simulink model "controller13_AIS"  (R2020b)
settings: Solver=FixedStepDiscrete  StartTime=0.0  StopTime=inf  RelTol=1e-3
values from neighbouring files (symbols this model uses):
  ctr = make_controller()    [setup_controller_with_functions.m]
  mdl = make_model(flight_time)    [setup_controller_with_functions.m]
  ukf_P0_flat = UKF.flatten_matrix(ukf_sys.P0)    [controller_setup_ukf.m]
  ukf_prediction_time = 0.015    [controller_setup_ukf.m]
  ukf_s0 = ukf_sys.s0    [controller_setup_ukf.m]
  ukf_sys = UKF.initialize_ukf_sys(rbt, mdl, ukf_params)    [controller_setup_ukf.m]
  ukf_use_prediction = 1    [controller_setup_ukf.m]
undefined symbols (not defined in the file or in its folder): ctr1, ctr2, DiscIntNeverNeededParam, flt, IO397, rbt1, rbt2, rsim1, rsim2, som, traj2
libraries: simulink x63, slrealtimeloglib x21, slrealtimetgmanagement x8, slrealtimeseriallib x5, speedgoatlib_fpga_analog_io x4, slrealtimeutilitieslib x3, dspfdesign x2, speedgoatlib_fpga x2, slrealtimeiplib x2, speedgoatlib_fpga_dio x1
(part 5 of 5)

== matlab function controller13_AIS/Adaptive Controller 1/somersault_phase ==
  data: som_phase output; time input; mdl parameter; som parameter
function som_phase  = fcn(time, mdl, som)
%#codegen

som_phase = 0;  % during a normal flight
if som.en
    if time > som.t_start + som.t_rise + som.t_acc + som.t_dcc + som.t_rec
        som_phase = 0;  % afterwards
    elseif time > som.t_start + som.t_rise + som.t_acc + som.t_dcc
        som_phase = 4;  % recovery
    elseif time > som.t_start + som.t_rise + som.t_acc
        som_phase = 3;  % rolling, second half.
    elseif time > som.t_start + som.t_rise
        som_phase = 2;  % rolling, first half.
    elseif time > som.t_start
        som_phase = 1;  % gaining altitude
    end
end

== matlab function controller13_AIS/Force//Torque to Trajectory Specs 1/nominal desired voltage/force to voltage flipping/MATLAB Function ==
  data: Vi input; Vo output; ctr1 parameter
function Vo = fcn(Vi,ctr1)
%old script
% if max(Vi)>mdl.max_v
%     Vo = Vi * mdl.max_v/max(Vi);
%     % scale down all votages if one exceeds the max limit.
% else
%     Vo = Vi;
% end

%new change (modify max_v to a vector so each DEA has its own max)
scale_down_ratio_vec = Vi ./ ctr1.safety.volt;
scale_down_ratio = max(scale_down_ratio_vec);
bool_scale_down = scale_down_ratio>1;

if bool_scale_down
   Vo = Vi/scale_down_ratio;
else
   Vo = Vi; 
end

== matlab function controller13_AIS/smothing 1/smoothing ==
  data: time input; out_amp output; amp input; amp2 input; som parameter
function out_amp  = fcn(time,amp,amp2,som)
%#codegen

alp = 1;
if time > som.t_start + som.t_rise + som.t_acc + som.t_dcc + som.t_rec
    alp = 1;  % afterwards
elseif time > som.t_start
    alp = som.filter.alp;
end
% set en = 0 if the robot goes out of the safe envelope.
out_amp = som.filter.alp*amp + (1-som.filter.alp)*amp2;

== matlab function controller13_AIS/Adaptive Controller 1/saturation ==
  data: x_roll input; X_roll output size=1; y_pitch input; z_yaw input; Y_pitch output size=1; Z_yaw output size=1; Th input; Force output size=1; rbt1 parameter; ctr1 parameter; som_phase input; som parameter
function [X_roll, Y_pitch, Z_yaw, Force] = fcn(x_roll, y_pitch, z_yaw, Th, rbt1, ctr1, som_phase, som)
%#codegen

X_roll = max(min(x_roll, ctr1.lim.taux), -ctr1.lim.taux);
%X_roll = x_roll;
Y_pitch = max(min(y_pitch, ctr1.lim.tauy), -ctr1.lim.tauy);
%Y_pitch = y_pitch;
Z_yaw = max(min(z_yaw, ctr1.lim.tauz), -ctr1.lim.tauz);

Force = Th*rbt1.m;

% F is already checked for saturation, but still needs to be converted into
% Newton

%% Roll torque management (somersault)
if som_phase == 2
    X_roll = som.roll_mag; % torque in SI
    Y_pitch = 0;  % to turn of the pitch control
elseif som_phase == 3
    X_roll = -som.roll_mag; % torque in SI
    Y_pitch = 0;  % to turn of the pitch control
end
    
%% Thrust management
% thrust is not controlled during the flipping maneuver (the output here will be overridden in the mapping).

== matlab function controller13_AIS/Force//Torque to Trajectory Specs 1/force//torque to module thrust/mapping scheme (flipping compataible) ==
  data: time input; module_f output; inputs input; rbt1 parameter; som parameter; mdl parameter
function module_f  = fcn(time, inputs, rbt1, som, mdl)

% somersault
if som.en
    if time > som.t_start + som.t_rise + som.t_acc + som.t_dcc+som.t_rec % after recovery
        %
    elseif time > som.t_start + som.t_rise + som.t_acc + som.t_dcc % recovery
        %inputs(1) = rbt.m*(mdl.g*(som.thrust_f+0.2));
    elseif time > som.t_start + som.t_rise % rolling, first half+second half.
        % priortize the roll torque and ensure non-negative forces.
        inputs(1) = 0;
    elseif time > som.t_start
        inputs(1) = rbt1.m*(mdl.g*som.thrust_f); % during the t rise.                
    end
end

% torque/thrust to unit force mapping
if rbt1.til == 0
    module_f = rbt1.Apinv * inputs(1:3); % original mapping
elseif rbt1.til > 0
    module_f = rbt1.A2inv * inputs;
else
    module_f = [0 0 0 0]';
end

% safety
if min(module_f) < 0
    module_f = module_f - min(module_f); % this ensure positive module forces
end

end

== matlab function controller13_AIS/Adaptive Controller 1/adaptive system/integrator/initial guess ==
  data: i_e input; int_e output; tor_off input; th_off input; tor_inte output; th_inte output; ctr1 parameter; rbt1 parameter; mdl parameter
function [int_e, tor_inte, th_inte] = fcn(i_e, tor_off, th_off, ctr1, rbt1, mdl)
%#codegen

tor_inte = zeros(3,1);
int_e    = zeros(4,1);

int_e(1) = i_e(1)+tor_off(1);
int_e(2) = i_e(2)+tor_off(2);
int_e(3) = i_e(3)+tor_off(3);
int_e(4) = i_e(4)+th_off;

tor_inte(1) = int_e(1)*ctr1.gain.ati*rbt1.ixx/mdl.g;
tor_inte(2) = int_e(2)*ctr1.gain.ati*rbt1.iyy/mdl.g;
tor_inte(3) = 0;

th_inte     = int_e(4)*ctr1.gain.ali;

== matlab function controller13_AIS/Phantom trigger/start at one ==
  data: time input; trigger output
function trigger = fcn(time)
%#codegen
trigger = 0;
if time > 1
   trigger = 1; 
end
if time > 2
   trigger = 0; 
end

== matlab function controller13_AIS/Measurement manager 1/safety check system/envelope check ==
  data: x input; en output; y input; z input; ctr1 parameter
function en  = fcn(x,y,z, ctr1)

if abs(x)>ctr1.safety.enableZone.xmax || abs(y)>ctr1.safety.enableZone.ymax || abs(z)>ctr1.safety.enableZone.zmax
    en = 0;
else
    en = 1;
end

end

== matlab function controller13_AIS/Dynamic Sim 1/conditioning ==
  data: Rout output; Rin input; eu output
function [Rout, eu]  = fcn(Rin)
%#codegen
Rm = [Rin(1:3)./norm(Rin(1:3)),Rin(4:6)./norm(Rin(4:6)),Rin(7:9)./norm(Rin(7:9))];
% conditioning on orthogonality.
Rout = [Rm(:,1);Rm(:,2);Rm(:,3)];

% euler angles
euy = asin(min(max(Rm(1,3),-1),1));
eux = atan2(-Rm(2,3),Rm(3,3));
euz = atan2(-Rm(1,2),Rm(1,1));
%euz=acos(min(max(Rm(1,1)/cos(euy),-1),1));
%eux=acos(min(max(Rm(3,3)/cos(euy),-1),1));
eu = [eux;euy;euz];
% not being very careful with singularities.

== matlab function controller13_AIS/Force//Torque to Trajectory Specs 1/nominal desired voltage/map_selection ==
  data: hover_map output; time input; mdl parameter; som parameter
function hover_map  = fcn(time, mdl, som)
%#codegen

hover_map = 1;  % during a normal flight
if som.en
    if time > som.t_start + som.t_rise + som.t_acc + som.t_dcc
        hover_map = 1;  % afterwards
    elseif time > som.t_start + som.t_rise
    %elseif time > som.t_start + som.t_rise 
        hover_map = 0;  % 
    end
end

== matlab function controller13_AIS/Dynamic Sim 1/rigid body dynamics sim ==
  data: dv output double size=3; mforces input double; dR output double size=9; dw output double size=3; v input; R input; w input; rbt1 parameter; mdl parameter; disturbance input; rsim1 parameter
function [dv, dR, dw]  = fcn(mforces,v,R,w,rbt1,mdl,disturbance, rsim1)
%#codegen

% noiseless
% no damping
% rbt_A_temp = [rbt.A; 0.015 -0.015 0.015 -0.015];
rbt_A_temp = rbt1.A2;
% inputs = rbt.A * mforces(:);
inputs = rbt_A_temp * mforces(:);
thrust = inputs(1);
% torque = [inputs(2);inputs(3);0];
torque = [inputs(2);inputs(3);inputs(4)];
%R = R(:);
%w = w(:);
dv = R(7:9)*thrust/rbt1.m - [0;0;mdl.g] + disturbance(1:3);

dw = diag([rsim1.rbt.ixx, rsim1.rbt.iyy, rsim1.rbt.izz]) \ ( (torque) - cross(w,diag([rsim1.rbt.ixx, rsim1.rbt.iyy, rsim1.rbt.izz])*w)+ disturbance(4:6) ) ;
dR1 = R(4:6)*w(3)-R(7:9)*w(2);
dR2 = R(7:9)*w(1)-R(1:3)*w(3);
dR3 = R(1:3)*w(2)-R(4:6)*w(1);
dR = [dR1;dR2;dR3];
%dv = zeros(3,1);
%dw = zeros(3,1);
%dR = zeros(9,1);

== matlab function controller13_AIS/Adaptive Controller 1/attitude and thrust controller/Yaw Controller/desired yaw ==
  data: t input; id input; rd_yaw output; ctr1 parameter; index output; mdl parameter
function [rd_yaw, index] = fcn(t,id,ctr1,mdl)

if ctr1.yaw.dy.en
    
    if id > 1
        t_cum = sum(ctr1.yaw.dy.duration(1:id-1))+sum(ctr1.yaw.dy.trans(1:id-1));
    else
        t_cum = 0;
    end

    if t > mdl.i_delay + t_cum && t <= mdl.i_delay + t_cum + ctr1.yaw.dy.duration(id)
        rd_yaw = ctr1.yaw.dy.angle(id);
    elseif t > mdl.i_delay + t_cum + ctr1.yaw.dy.duration(id) && t < mdl.i_delay + t_cum + ctr1.yaw.dy.duration(id) + ctr1.yaw.dy.trans(id)
        rd_yaw = ctr1.yaw.dy.angle(id) + (ctr1.yaw.dy.angle(id+1)-ctr1.yaw.dy.angle(id))/ctr1.yaw.dy.trans(id)*(t-mdl.i_delay-t_cum-ctr1.yaw.dy.duration(id));
    elseif t >= mdl.i_delay + t_cum + ctr1.yaw.dy.duration(id) + ctr1.yaw.dy.trans(id)
        rd_yaw = ctr1.yaw.dy.angle(id+1);
        id = id + 1;
    else
        rd_yaw = 0;
    end

else
    
    rd_yaw = ctr1.setpoint.yaw;
    
end

index = id;
    
end

== matlab function controller13_AIS/Measurement manager 1/safety check system/voltage check ==
  data: voltage input; en output; ctr1 parameter
function en  = fcn(voltage, ctr1)

if sum(voltage>ctr1.safety.volt) > 0
    en = 0;
else
    en = 1;
end

end

== matlab function controller13_AIS/Measurement manager 1/envelope//voltage check ==
  data: x input; keep_flying output size=1; y input; z input; ctr1 parameter
function keep_flying  = fcn(x,y,z,ctr1)

if abs(x)>ctr1.safety.land.xmax || abs(y)>ctr1.safety.land.ymax || abs(z)>ctr1.safety.land.zmax
    keep_flying = 0;
% elseif voltage(1) > ctr.safety.land.volt
%     keep_flying = 0;    
else
    keep_flying = 1;
end

end

== matlab function controller13_AIS/Measurement manager 1/MATLAB Function ==
  data: keep_flying input; landing_in input; landing_out output size=1; cum_in input; cum_out output size=1; ctr1 parameter; mdl parameter
function [landing_out, cum_out] = fcn(keep_flying, landing_in, cum_in, ctr1, mdl)

if keep_flying == 0
    cum_out = cum_in + mdl.T;
else
    cum_out = 0;
end

if cum_out > ctr1.safety.land.T || landing_in == 1
    landing_out = 1;
else 
    landing_out = 0;
end

end

== matlab function controller13_AIS/Measurement manager 1/voltage check ==
  data: voltage input; keep_flying output size=1; ctr1 parameter
function keep_flying  = fcn(voltage, ctr1)

% if voltage(1)>ctr.safety.land.volt || voltage(2)>ctr.safety.land.volt || voltage(3)>ctr.safety.land.volt || voltage(4)>ctr.safety.land.volt

if sum(voltage>ctr1.safety.land.volt)>0
    keep_flying = 0;
else
    keep_flying = 1;
end

end

== matlab function controller13_AIS/Measurement manager 1/safety check system/MATLAB Function ==
  data: keep_flying input; en_in input; en_out output size=1; cum_in input; cum_out output size=1; ctr1 parameter; mdl parameter
function [en_out, cum_out] = fcn(keep_flying, en_in, cum_in, ctr1, mdl)

if keep_flying == 0
    cum_out = cum_in + mdl.T;
else
    cum_out = 0;
end

if cum_out > ctr1.safety.T || en_in == 0
    en_out = 0;
else 
    en_out = 1;
end

end

== matlab function controller13_AIS/MATLAB Function ==
  data: u input; y output
function y = fcn(u)

y = u;

== matlab function controller13_AIS/Adaptive Controller 1/attitude and thrust controller/External Torque Observer ==
  data: omega input; omega_hat output; torque_x input; torque_y input; torque_z input; ext_torque_hat input; omega_hat input; time input; ext_torque_hat output; ctr1 parameter; rbt1 parameter; mdl parameter
function [omega_hat, ext_torque_hat] = fcn(omega, torque_x, torque_y, torque_z, ext_torque_hat, omega_hat, time, ctr1, rbt1, mdl)
    
omega_hat           = omega_hat(:);
ext_torque_hat      = ext_torque_hat(:);
J                   = diag([rbt1.ixx, rbt1.iyy, rbt1.izz]);
omega_cross_J_omega = cross(omega, J*omega);
x_hat_curr          = diag(ctr1.torque_obs.state_scaling)*[omega_hat(:); ext_torque_hat(:)];

% til = 20;

if rbt1.til == 0
    u              = diag(ctr1.torque_obs.input_scaling)*[torque_x - omega_cross_J_omega(1); torque_y - omega_cross_J_omega(2)];
    y              = diag(ctr1.torque_obs.meas_scaling)*omega(1:2); 
    x_hat_pred     = ctr1.torque_obs.A*x_hat_curr + ctr1.torque_obs.B(:, 1:2)*u; 
    x_hat_next     = diag(ctr1.torque_obs.out_scaling)*(x_hat_pred + ctr1.torque_obs.L*(y - ctr1.torque_obs.C*x_hat_pred));
    omega_hat      = x_hat_next(1:2,1);
    ext_torque_hat = x_hat_next(3:4,1);
    if time < mdl.i_delay
        omega_hat      = zeros(2,1);
        ext_torque_hat = zeros(2,1);
    end
else
    u              = diag(ctr1.torque_obs.input_scaling)*[torque_x - omega_cross_J_omega(1); torque_y - omega_cross_J_omega(2); torque_z - omega_cross_J_omega(3)];
    y              = diag(ctr1.torque_obs.meas_scaling)*omega(1:3); 
    x_hat_pred     = ctr1.torque_obs.A*x_hat_curr + ctr1.torque_obs.B(:, 1:3)*u; 
    x_hat_next     = diag(ctr1.torque_obs.out_scaling)*(x_hat_pred + ctr1.torque_obs.L*(y - ctr1.torque_obs.C*x_hat_pred));
    omega_hat      = x_hat_next(1:3,1);
    ext_torque_hat = x_hat_next(4:6,1);
    if time < mdl.i_delay
        omega_hat      = zeros(3,1);
        ext_torque_hat = zeros(3,1);
    end
end



end

== matlab function controller13_AIS/Adaptive Controller 2/adaptive setpoint rd ==
  data: rd output; rd_d output; rd_dd output; rd_ddd output; rd_dddd output; time input; r input; r_d input; landing input; som_ph input; id_in input; ctr2 parameter; som parameter; mdl parameter; traj2 parameter; id_out output
function [rd,rd_d,rd_dd,rd_ddd,rd_dddd,id_out] = fcn(time, r, r_d, landing, som_ph, id_in, ctr2, som, mdl, traj2)
%#codegen

rd = [ctr2.setpoint.x; ctr2.setpoint.y; ctr2.setpoint.z];
rd_d = zeros(3,1);
rd_dd = zeros(3,1);
rd_ddd = zeros(3,1);
rd_dddd = zeros(3,1);

if time <= mdl.i_delay+0.1
    rd_z = ctr2.takeoff.height;
    rd   = [ctr2.setpoint.x; ctr2.setpoint.y; rd_z];
end

% takeoff
if ctr2.takeoff.en
    if time > mdl.i_delay+0.1 && time < (mdl.i_delay+0.1+ctr2.takeoff.time)
        
        % rd_z (desired position)
        rd_z = ctr2.takeoff.height + (((ctr2.setpoint.z-ctr2.takeoff.height)/ctr2.takeoff.time)*(time-mdl.i_delay-0.1));
        if rd_z > ctr2.setpoint.z
            rd_z = ctr2.setpoint.z;
        end
        rd   = [ctr2.setpoint.x; ctr2.setpoint.y; rd_z];
        
        % rd_d_z (desired velocity)
        rd_d_z = ((ctr2.setpoint.z-ctr2.takeoff.height)/ctr2.takeoff.time);
        rd_d   = [rd_d(1); rd_d(2); rd_d_z];
        
    end
end

% planned landing 
if ctr2.landing.en
    if time > (mdl.rt-ctr2.landing.time)
        
        % rd_z (desired position)
        rd_z = ctr2.setpoint.z-(((ctr2.setpoint.z-ctr2.landing.height)/ctr2.landing.time)*(time-mdl.rt+ctr2.landing.time));
        if rd_z < ctr2.landing.height
            rd_z = ctr2.landing.height;
        end
        rd   = [ctr2.setpoint.x; ctr2.setpoint.y; rd_z];
        
        % rd_d_z (desired velocity)
        rd_d_z = (ctr2.landing.height-ctr2.setpoint.z)/ctr2.landing.time;
        rd_d   = [rd_d(1); rd_d(2); rd_d_z];
        
    end
end

% forced landing
if landing
    rd_z = 0.02;
    rd   = [ctr2.setpoint.x; ctr2.setpoint.y; rd_z];
end


% somersault
if som.en
    if time > som.t_start + som.t_rise + som.t_acc + som.t_dcc + som.t_rec
        % % afterwards 
        %dt = som.t_start + som.t_rise + som.t_acc + som.t_dcc + som.t_rec - time;
        %rd = rd + dt*(r-rd);
    elseif time > som.t_start + som.t_rise + som.t_acc + som.t_dcc
        % recovery
        dt = som.t_start + som.t_rise + som.t_acc + som.t_dcc + som.t_rec - time;
        rd = rd + (dt/som.t_rec)*(r-rd);
        rd_d = rd_d + 0.5*(dt/som.t_rec)*(r_d-rd_d);
        rd(1) = min(max(rd(1),-0.25),0.25); % 25 cm envelope
        rd(2) = min(max(rd(2),-0.25),0.25); % 25 cm envelope
        rd(3) = max(rd(3),0.02); % min altitude setpoint.
    end
end

% update id for predefined trajectory
id      = floor(id_in);
id_out  = id_in + 1;

% use predefined trajectory
if traj2.en
    rd      = traj2.origin + traj2.rd(1:3,id);
    rd_d    = traj2.rd_d(1:3,id);
    rd_dd   = traj2.rd_dd(1:3,id);
    rd_ddd  = traj2.rd_ddd(1:3,id);
    rd_dddd = traj2.rd_dddd(1:3,id);
end



end

== matlab function controller13_AIS/Adaptive Controller 1/attitude and thrust controller/Yaw Controller/MATLAB Function ==
  data: torq_ext input; torq_z input; torq_z output; ctr1 parameter; rbt1 parameter
function torq_z = fcn(torq_ext,torq_z,ctr1, rbt1)

% if rbt1.til > 0
%     if ctr1.yaw.dy.en == 0
%         torq_z = torq_z - torq_ext(3) * ctr1.torque_obs.factor.z;
%     end
% end

end

== matlab function controller13_AIS/Adaptive Controller 2/adaptive system/integrator/initial guess ==
  data: i_e input; int_e output; tor_off input; th_off input; tor_inte output; th_inte output; ctr2 parameter; rbt2 parameter; mdl parameter
function [int_e, tor_inte, th_inte] = fcn(i_e, tor_off, th_off, ctr2, rbt2, mdl)
%#codegen

tor_inte = zeros(3,1);
int_e    = zeros(4,1);

int_e(1) = i_e(1)+tor_off(1);
int_e(2) = i_e(2)+tor_off(2);
int_e(3) = i_e(3)+tor_off(3);
int_e(4) = i_e(4)+th_off;

tor_inte(1) = int_e(1)*ctr2.gain.ati*rbt2.ixx/mdl.g;
tor_inte(2) = int_e(2)*ctr2.gain.ati*rbt2.iyy/mdl.g;
tor_inte(3) = 0;

th_inte     = int_e(4)*ctr2.gain.ali;

== matlab function controller13_AIS/Adaptive Controller 2/attitude and thrust controller/Attitude Controleller ==
  data: r input; torque_x output size=1; r_dot input; r_dotdot input; R input; Omega input; rd input; rd_d input; rd_dd input; rd_ddd input; rd_dddd input; int_e input; ext_torq input; ctr2 parameter; rbt2 parameter; torque_y output size=1; torque_z output size=1; att_e output size=3; mdl parameter
 function [torque_x, torque_y, torque_z, att_e] = fcn(r, r_dot, r_dotdot, R, Omega, rd,rd_d,rd_dd,rd_ddd,rd_dddd, int_e, ext_torq, ctr2, rbt2, mdl)
%#codegen

%% init
R11 = R(1);
R12 = R(2);
R13 = R(3);
R21 = R(4);
R22 = R(5);
R23 = R(6);
R31 = R(7);
R32 = R(8);
R33 = R(9);
R1 = [R11; R21; R31];     % unit (column) vector
R2 = [R12; R22; R32];
R3 = [R13; R23; R33];
wx = Omega(1);
wy = Omega(2);
wz = Omega(3);

Dr = r-rd;
Dr_dot = r_dot-rd_d;

torque_x = -dot(R2,rd_dddd) - ...
    ctr2.gain.at3*( mdl.g*wx+dot(R2,rd_ddd) ) - ...
    ctr2.gain.at2*( dot(R2,mdl.g*[0;0;1]+rd_dd) ) + ...
    ctr2.gain.at1*( dot(R2,Dr_dot) ) + ...
    ctr2.gain.at0*( dot(R2,Dr) ) + ...
    ctr2.gain.ati*( int_e(1) );
torque_x = torque_x*rbt2.ixx/mdl.g - ext_torq(1)*ctr2.torque_obs.factor.x;

torque_y = dot(R1,rd_dddd) - ...
    ctr2.gain.at3*( mdl.g*wy-dot(R1,rd_ddd) ) - ...
    ctr2.gain.at2*( dot(R1,-mdl.g*[0;0;1]-rd_dd) ) - ...
    ctr2.gain.at1*( dot(R1,Dr_dot) ) - ...
    ctr2.gain.at0*( dot(R1,Dr) ) + ...
    ctr2.gain.ati*( int_e(2) );

torque_y = torque_y*rbt2.iyy/mdl.g - ext_torq(2)*ctr2.torque_obs.factor.y;

torque_z = 0;           % no yaw control

att_e = -[-dot(R2,Dr);dot(R1,Dr);0];

== matlab function controller13_AIS/Adaptive Controller 1/observer/Rotaion/Rotation Matrix1 ==
  data: R input; Rdot input; w output
function w  = fcn(R,Rdot)
%#codegen
w = zeros(3,1);
w(1) = R(3)*Rdot(2) + R(6)*Rdot(5) + R(9)*Rdot(8);
w(2) = R(1)*Rdot(3) + R(4)*Rdot(6) + R(7)*Rdot(9);
w(3) = R(2)*Rdot(1) + R(5)*Rdot(4) + R(8)*Rdot(7);

% w = R^T * dot(R)

end

== matlab function controller13_AIS/Adaptive Controller 2/attitude and thrust controller/External Torque Observer ==
  data: omega input; omega_hat output; torque_x input; torque_y input; torque_z input; ext_torque_hat input; omega_hat input; time input; ext_torque_hat output; ctr2 parameter; rbt2 parameter; mdl parameter
function [omega_hat, ext_torque_hat] = fcn(omega, torque_x, torque_y, torque_z, ext_torque_hat, omega_hat, time, ctr2, rbt2, mdl)
    
omega_hat           = omega_hat(:);
ext_torque_hat      = ext_torque_hat(:);
J                   = diag([rbt2.ixx, rbt2.iyy, rbt2.izz]);
omega_cross_J_omega = cross(omega, J*omega);
x_hat_curr          = diag(ctr2.torque_obs.state_scaling)*[omega_hat(:); ext_torque_hat(:)];

% til = 20;

if rbt2.til == 0
    u              = diag(ctr2.torque_obs.input_scaling)*[torque_x - omega_cross_J_omega(1); torque_y - omega_cross_J_omega(2)];
    y              = diag(ctr2.torque_obs.meas_scaling)*omega(1:2); 
    x_hat_pred     = ctr2.torque_obs.A*x_hat_curr + ctr2.torque_obs.B(:, 1:2)*u; 
    x_hat_next     = diag(ctr2.torque_obs.out_scaling)*(x_hat_pred + ctr2.torque_obs.L*(y - ctr2.torque_obs.C*x_hat_pred));
    omega_hat      = x_hat_next(1:2,1);
    ext_torque_hat = x_hat_next(3:4,1);
    if time < mdl.i_delay
        omega_hat      = zeros(2,1);
        ext_torque_hat = zeros(2,1);
    end
else
    u              = diag(ctr2.torque_obs.input_scaling)*[torque_x - omega_cross_J_omega(1); torque_y - omega_cross_J_omega(2); torque_z - omega_cross_J_omega(3)];
    y              = diag(ctr2.torque_obs.meas_scaling)*omega(1:3); 
    x_hat_pred     = ctr2.torque_obs.A*x_hat_curr + ctr2.torque_obs.B(:, 1:3)*u; 
    x_hat_next     = diag(ctr2.torque_obs.out_scaling)*(x_hat_pred + ctr2.torque_obs.L*(y - ctr2.torque_obs.C*x_hat_pred));
    omega_hat      = x_hat_next(1:3,1);
    ext_torque_hat = x_hat_next(4:6,1);
    if time < mdl.i_delay
        omega_hat      = zeros(3,1);
        ext_torque_hat = zeros(3,1);
    end
end



end

== matlab function controller13_AIS/Adaptive Controller 2/attitude and thrust controller/Thrust Controller ==
  data: r input; F output size=1; r_dot input; r_dotdot input; R input; Omega input; rd input; rd_d input; rd_dd input; rd_ddd input; rd_dddd input; int_e input; mdl parameter; alt_e output size=1; ctr2 parameter
function [F, alt_e] = fcn(r, r_dot, r_dotdot, R, Omega, rd,rd_d,rd_dd,rd_ddd,rd_dddd, int_e, mdl, ctr2)
%#codegen

%% init
R11 = R(1);
R12 = R(2);
R13 = R(3);
R21 = R(4);
R22 = R(5);
R23 = R(6);
R31 = R(7);
R32 = R(8);
R33 = R(9);

% feedforward
% -> (0m, 0) -> (0.1m, 0.2)
ffwd = mdl.g * max(0,(rd(3)*1.25-ctr2.takeoff.height));

F = rd_dd(3) - ctr2.gain.al1*( r_dot(3)-rd_d(3) ) - ctr2.gain.al0*( r(3)-rd(3) );
% F = 0 - ctr.gain.al1*( r_dot(3)) - ctr.gain.al0*( r(3)-ctr.setpoint.z );
F = mdl.g + F + ctr2.gain.ali*int_e(4) + ffwd; % g + control + integral + feedforward
F = F/R33;
F = max(min(F, mdl.g+4), mdl.g-4.0); % during hovering.

alt_e = -( r(3)-rd(3) )/R33;
% alt_e = -( r(3)- ctr.setpoint.z )/R33;
end

== matlab function controller13_AIS/Adaptive Controller 2/attitude and thrust controller/Yaw Controller/MATLAB Function ==
  data: torq_ext input; torq_z input; torq_z output; ctr2 parameter; rbt2 parameter
function torq_z = fcn(torq_ext,torq_z,ctr2, rbt2)

if rbt2.til > 0
    if ctr2.yaw.dy.en == 0
%         torq_z = torq_z - torq_ext(3) * ctr2.torque_obs.factor.z;
    end
else
    torq_z = torq_z;
end

end

== matlab function controller13_AIS/Adaptive Controller 2/attitude and thrust controller/Yaw Controller/desired yaw ==
  data: t input; id input; rd_yaw output; ctr2 parameter; index output; mdl parameter
function [rd_yaw, index] = fcn(t,id,ctr2,mdl)

if ctr2.yaw.dy.en
    
    if id > 1
        t_cum = sum(ctr2.yaw.dy.duration(1:id-1))+sum(ctr2.yaw.dy.trans(1:id-1));
    else
        t_cum = 0;
    end

    if t > mdl.i_delay + t_cum && t <= mdl.i_delay + t_cum + ctr2.yaw.dy.duration(id)
        rd_yaw = ctr2.yaw.dy.angle(id);
    elseif t > mdl.i_delay + t_cum + ctr2.yaw.dy.duration(id) && t < mdl.i_delay + t_cum + ctr2.yaw.dy.duration(id) + ctr2.yaw.dy.trans(id)
        rd_yaw = ctr2.yaw.dy.angle(id) + (ctr2.yaw.dy.angle(id+1)-ctr2.yaw.dy.angle(id))/ctr2.yaw.dy.trans(id)*(t-mdl.i_delay-t_cum-ctr2.yaw.dy.duration(id));
    elseif t >= mdl.i_delay + t_cum + ctr2.yaw.dy.duration(id) + ctr2.yaw.dy.trans(id)
        rd_yaw = ctr2.yaw.dy.angle(id+1);
        id = id + 1;
    else
        rd_yaw = 0;
    end

else
    
    rd_yaw = ctr2.setpoint.yaw;
    
end

index = id;
    
end

== matlab function controller13_AIS/Adaptive Controller 2/observer/Rotaion/Rotation Matrix ==
  data: euler_angles input; R output
function R = fcn(euler_angles)
%#codegen

eu_x = euler_angles(1);
eu_y = euler_angles(2);
eu_z = euler_angles(3);

R = [cos(eu_y)*cos(eu_z); -cos(eu_y)*sin(eu_z); sin(eu_y); ...
    cos(eu_x)*sin(eu_z)+sin(eu_x)*sin(eu_y)*cos(eu_z); cos(eu_x)*cos(eu_z)-sin(eu_x)*sin(eu_y)*sin(eu_z); -sin(eu_x)*cos(eu_y); ...
    sin(eu_x)*sin(eu_z)-cos(eu_x)*sin(eu_y)*cos(eu_z); sin(eu_x)*cos(eu_z)+cos(eu_x)*sin(eu_y)*sin(eu_z); cos(eu_x)*cos(eu_y)];
% R is 1x9

== matlab function controller13_AIS/Adaptive Controller 2/observer/Rotaion/Rotation Matrix1 ==
  data: R input; Rdot input; w output
function w  = fcn(R,Rdot)
%#codegen
w = zeros(3,1);
w(1) = R(3)*Rdot(2) + R(6)*Rdot(5) + R(9)*Rdot(8);
w(2) = R(1)*Rdot(3) + R(4)*Rdot(6) + R(7)*Rdot(9);
w(3) = R(2)*Rdot(1) + R(5)*Rdot(4) + R(8)*Rdot(7);

== matlab function controller13_AIS/Adaptive Controller 1/attitude and thrust controller/Attitude Controleller ==
  data: r input; torque_x output size=1; r_dot input; r_dotdot input; R input; Omega input; rd input; rd_d input; rd_dd input; rd_ddd input; rd_dddd input; int_e input; ext_torq input; ctr1 parameter; rbt1 parameter; torque_y output size=1; torque_z output size=1; att_e output size=3; mdl parameter
 function [torque_x, torque_y, torque_z, att_e] = fcn(r, r_dot, r_dotdot, R, Omega, rd,rd_d,rd_dd,rd_ddd,rd_dddd, int_e, ext_torq, ctr1, rbt1, mdl)
%#codegen

%% init
R11 = R(1);
R12 = R(2);
R13 = R(3);
R21 = R(4);
R22 = R(5);
R23 = R(6);
R31 = R(7);
R32 = R(8);
R33 = R(9);
R1 = [R11; R21; R31];     % unit (column) vector
R2 = [R12; R22; R32];
R3 = [R13; R23; R33];
wx = Omega(1);
wy = Omega(2);
wz = Omega(3);

Dr = r-rd;
Dr_dot = r_dot-rd_d;

torque_x = -dot(R2,rd_dddd) - ...
    ctr1.gain.at3*( mdl.g*wx+dot(R2,rd_ddd) ) - ...
    ctr1.gain.at2*( dot(R2,mdl.g*[0;0;1]+rd_dd) ) + ...
    ctr1.gain.at1*( dot(R2,Dr_dot) ) + ...
    ctr1.gain.at0*( dot(R2,Dr) ) + ...
    ctr1.gain.ati*( int_e(1) );
torque_x = torque_x*rbt1.ixx/mdl.g - ext_torq(1)*ctr1.torque_obs.factor.x;

torque_y = dot(R1,rd_dddd) - ...
    ctr1.gain.at3*( mdl.g*wy-dot(R1,rd_ddd) ) - ...
    ctr1.gain.at2*( dot(R1,-mdl.g*[0;0;1]-rd_dd) ) - ...
    ctr1.gain.at1*( dot(R1,Dr_dot) ) - ...
    ctr1.gain.at0*( dot(R1,Dr) ) + ...
    ctr1.gain.ati*( int_e(2) );

torque_y = torque_y*rbt1.iyy/mdl.g - ext_torq(2)*ctr1.torque_obs.factor.y;

torque_z = 0;           % no yaw control

att_e = -[-dot(R2,Dr);dot(R1,Dr);0];

== matlab function controller13_AIS/Adaptive Controller 2/saturation ==
  data: x_roll input; X_roll output size=1; y_pitch input; z_yaw input; Y_pitch output size=1; Z_yaw output size=1; Th input; Force output size=1; rbt2 parameter; ctr2 parameter; som_phase input; som parameter
function [X_roll, Y_pitch, Z_yaw, Force] = fcn(x_roll, y_pitch, z_yaw, Th, rbt2, ctr2, som_phase, som)
%#codegen

X_roll = max(min(x_roll, ctr2.lim.taux), -ctr2.lim.taux);
%X_roll = x_roll;
Y_pitch = max(min(y_pitch, ctr2.lim.tauy), -ctr2.lim.tauy);
%Y_pitch = y_pitch;
Z_yaw = max(min(z_yaw, ctr2.lim.tauz), -ctr2.lim.tauz);

Force = Th*rbt2.m;

% F is already checked for saturation, but still needs to be converted into
% Newton

%% Roll torque management (somersault)
if som_phase == 2
    X_roll = som.roll_mag; % torque in SI
    Y_pitch = 0;  % to turn of the pitch control
elseif som_phase == 3
    X_roll = -som.roll_mag; % torque in SI
    Y_pitch = 0;  % to turn of the pitch control
end
    
%% Thrust management
% thrust is not controlled during the flipping maneuver (the output here will be overridden in the mapping).

== matlab function controller13_AIS/Adaptive Controller 2/somersault_phase ==
  data: som_phase output; time input; mdl parameter; som parameter
function som_phase  = fcn(time, mdl, som)
%#codegen

som_phase = 0;  % during a normal flight
if som.en
    if time > som.t_start + som.t_rise + som.t_acc + som.t_dcc + som.t_rec
        som_phase = 0;  % afterwards
    elseif time > som.t_start + som.t_rise + som.t_acc + som.t_dcc
        som_phase = 4;  % recovery
    elseif time > som.t_start + som.t_rise + som.t_acc
        som_phase = 3;  % rolling, second half.
    elseif time > som.t_start + som.t_rise
        som_phase = 2;  % rolling, first half.
    elseif time > som.t_start
        som_phase = 1;  % gaining altitude
    end
end

== matlab function controller13_AIS/Dynamic Sim 2/conditioning ==
  data: Rout output; Rin input; eu output
function [Rout, eu]  = fcn(Rin)
%#codegen
Rm = [Rin(1:3)./norm(Rin(1:3)),Rin(4:6)./norm(Rin(4:6)),Rin(7:9)./norm(Rin(7:9))];
% conditioning on orthogonality.
Rout = [Rm(:,1);Rm(:,2);Rm(:,3)];

% euler angles
euy = asin(min(max(Rm(1,3),-1),1));
eux = atan2(-Rm(2,3),Rm(3,3));
euz = atan2(-Rm(1,2),Rm(1,1));
%euz=acos(min(max(Rm(1,1)/cos(euy),-1),1));
%eux=acos(min(max(Rm(3,3)/cos(euy),-1),1));
eu = [eux;euy;euz];
% not being very careful with singularities.

== matlab function controller13_AIS/Dynamic Sim 2/rigid body dynamics sim ==
  data: dv output double size=3; mforces input double; dR output double size=9; dw output double size=3; v input; R input; w input; rbt2 parameter; mdl parameter; disturbance input; rsim2 parameter
function [dv, dR, dw]  = fcn(mforces,v,R,w,rbt2,mdl,disturbance, rsim2)
%#codegen

% noiseless
% no damping
% rbt_A_temp = [rbt.A; 0.015 -0.015 0.015 -0.015];
rbt_A_temp = rbt2.A2;
% inputs = rbt.A * mforces(:);
inputs = rbt_A_temp * mforces(:);
thrust = inputs(1);
% torque = [inputs(2);inputs(3);0];
torque = [inputs(2);inputs(3);inputs(4)];
%R = R(:);
%w = w(:);
dv = R(7:9)*thrust/rbt2.m - [0;0;mdl.g] + disturbance(1:3);

dw = diag([rsim2.rbt.ixx, rsim2.rbt.iyy, rsim2.rbt.izz]) \ ( (torque) - 1e-7*w - cross(w,diag([rsim2.rbt.ixx, rsim2.rbt.iyy, rsim2.rbt.izz])*w)+ disturbance(4:6) ) ;
dR1 = R(4:6)*w(3)-R(7:9)*w(2);
dR2 = R(7:9)*w(1)-R(1:3)*w(3);
dR3 = R(1:3)*w(2)-R(4:6)*w(1);
dR = [dR1;dR2;dR3];
%dv = zeros(3,1);
%dw = zeros(3,1);
%dR = zeros(9,1);

== matlab function controller13_AIS/Force//Torque to Trajectory Specs 2/force//torque to module thrust/mapping scheme (flipping compataible) ==
  data: time input; module_f output; inputs input; rbt2 parameter; som parameter; mdl parameter
function module_f  = fcn(time, inputs, rbt2, som, mdl)

% somersault
if som.en
    if time > som.t_start + som.t_rise + som.t_acc + som.t_dcc+som.t_rec % after recovery
        %
    elseif time > som.t_start + som.t_rise + som.t_acc + som.t_dcc % recovery
        %inputs(1) = rbt.m*(mdl.g*(som.thrust_f+0.2));
    elseif time > som.t_start + som.t_rise % rolling, first half+second half.
        % priortize the roll torque and ensure non-negative forces.
        inputs(1) = 0;
    elseif time > som.t_start
        inputs(1) = rbt2.m*(mdl.g*som.thrust_f); % during the t rise.                
    end
end

% torque/thrust to unit force mapping
if rbt2.til == 0
    module_f = rbt2.Apinv * inputs(1:3); % original mapping
elseif rbt2.til > 0
    module_f = rbt2.A2inv * inputs;
else
    module_f = [0 0 0 0]';
end

% safety
if min(module_f) < 0
    module_f = module_f - min(module_f); % this ensure positive module forces
end

end

== matlab function controller13_AIS/Force//Torque to Trajectory Specs 2/nominal desired voltage/force to voltage (hovering) /MATLAB Function ==
  data: Vi input; Vo output; mdl parameter; ctr2 parameter
function Vo = fcn(Vi,mdl,ctr2)
%old script
% if max(Vi)>mdl.max_v
%     Vo = Vi * mdl.max_v/max(Vi);
%     % scale down all votages if one exceeds the max limit.
% else
%     Vo = Vi;
% end

%new change (modify max_v to a vector so each DEA has its own max)
% scale_down_ratio_vec = Vi ./ mdl.max_v_vec;
% scale_down_ratio = max(scale_down_ratio_vec);
% bool_scale_down = scale_down_ratio>1;
% 
% if bool_scale_down
%    Vo = Vi/scale_down_ratio;
% else
%    Vo = Vi; 
% end

min_v_vec = mdl.hovering_vec -150;
scale_down_ratio_vec = (Vi-min_v_vec)./(ctr2.safety.volt-min_v_vec);

scale_down_ratio = max(scale_down_ratio_vec);
bool_scale_down = scale_down_ratio>1;

if bool_scale_down
    Vo = min_v_vec + (Vi - min_v_vec)./scale_down_ratio;	
else
	  Vo = Vi; 
end


%extra layer of safety
for i=1:length(Vo)
	Vo(i) = min(Vo(i),ctr2.safety.volt(i));
end

== matlab function controller13_AIS/Force//Torque to Trajectory Specs 2/nominal desired voltage/force to voltage flipping/MATLAB Function ==
  data: Vi input; Vo output; ctr2 parameter
function Vo = fcn(Vi,ctr2)
%old script
% if max(Vi)>mdl.max_v
%     Vo = Vi * mdl.max_v/max(Vi);
%     % scale down all votages if one exceeds the max limit.
% else
%     Vo = Vi;
% end

%new change (modify max_v to a vector so each DEA has its own max)
scale_down_ratio_vec = Vi ./ ctr2.safety.volt;
scale_down_ratio = max(scale_down_ratio_vec);
bool_scale_down = scale_down_ratio>1;

if bool_scale_down
   Vo = Vi/scale_down_ratio;
else
   Vo = Vi; 
end

== matlab function controller13_AIS/Force//Torque to Trajectory Specs 2/nominal desired voltage/map_selection ==
  data: hover_map output; time input; mdl parameter; som parameter
function hover_map  = fcn(time, mdl, som)
%#codegen

hover_map = 1;  % during a normal flight
if som.en
    if time > som.t_start + som.t_rise + som.t_acc + som.t_dcc
        hover_map = 1;  % afterwards
    elseif time > som.t_start + som.t_rise
    %elseif time > som.t_start + som.t_rise 
        hover_map = 0;  % 
    end
end

== matlab function controller13_AIS/MATLAB Function1 ==
  data: u input; y output
function y = fcn(u)

y = u;

== matlab function controller13_AIS/Measurement manager 2/MATLAB Function ==
  data: keep_flying input; landing_in input; landing_out output size=1; cum_in input; cum_out output size=1; ctr2 parameter; mdl parameter
function [landing_out, cum_out] = fcn(keep_flying, landing_in, cum_in, ctr2, mdl)

if keep_flying == 0
    cum_out = cum_in + mdl.T;
else
    cum_out = 0;
end

if cum_out > ctr2.safety.land.T || landing_in == 1
    landing_out = 1;
else 
    landing_out = 0;
end

end

== matlab function controller13_AIS/Measurement manager 2/envelope//voltage check ==
  data: x input; keep_flying output size=1; y input; z input; ctr2 parameter
function keep_flying  = fcn(x,y,z,ctr2)

if abs(x)>ctr2.safety.land.xmax || abs(y)>ctr2.safety.land.ymax || abs(z)>ctr2.safety.land.zmax
    keep_flying = 0;
% elseif voltage(1) > ctr.safety.land.volt
%     keep_flying = 0;    
else
    keep_flying = 1;
end

end

== matlab function controller13_AIS/Measurement manager 2/safety check system/MATLAB Function ==
  data: keep_flying input; en_in input; en_out output size=1; cum_in input; cum_out output size=1; ctr2 parameter; mdl parameter
function [en_out, cum_out] = fcn(keep_flying, en_in, cum_in, ctr2, mdl)

if keep_flying == 0
    cum_out = cum_in + mdl.T;
else
    cum_out = 0;
end

if cum_out > ctr2.safety.T || en_in == 0
    en_out = 0;
else 
    en_out = 1;
end

end

== matlab function controller13_AIS/Measurement manager 2/safety check system/envelope check ==
  data: x input; en output; y input; z input; ctr2 parameter
function en  = fcn(x,y,z, ctr2)

if abs(x)>ctr2.safety.enableZone.xmax || abs(y)>ctr2.safety.enableZone.ymax || abs(z)>ctr2.safety.enableZone.zmax
    en = 0;
else
    en = 1;
end

end

== matlab function controller13_AIS/Measurement manager 2/safety check system/landing condition/landing_cond ==
  data: alt input; en output; time_cond input; ctr2 parameter
function en = fcn(alt,time_cond,ctr2)
%#codegen
if ( (time_cond<0) | (alt>ctr2.landing.height) )
    en = 1;
else
    en = 0;
end
en=1;
end
% this lands the robot if the flight time is more than mdl.i_delay+2 and
% the robot is still on the ground.

== matlab function controller13_AIS/Measurement manager 2/safety check system/voltage check ==
  data: voltage input; en output; ctr2 parameter
function en  = fcn(voltage, ctr2)

if sum(voltage>ctr2.safety.volt) > 0
    en = 0;
else
    en = 1;
end

end

== matlab function controller13_AIS/Measurement manager 2/voltage check ==
  data: voltage input; keep_flying output size=1; ctr2 parameter
function keep_flying  = fcn(voltage, ctr2)

% if voltage(1)>ctr.safety.land.volt || voltage(2)>ctr.safety.land.volt || voltage(3)>ctr.safety.land.volt || voltage(4)>ctr.safety.land.volt

if sum(voltage>ctr2.safety.land.volt)>0
    keep_flying = 0;
else
    keep_flying = 1;
end

end

== matlab function controller13_AIS/Vicon Measurements/MATLAB Function ==
  data: u input; y output
function y = fcn(u)

y = u;

== matlab function controller13_AIS/smothing 2/smoothing ==
  data: time input; out_amp output; amp input; amp2 input; som parameter
function out_amp  = fcn(time,amp,amp2,som)
%#codegen

alp = 1;
if time > som.t_start + som.t_rise + som.t_acc + som.t_dcc + som.t_rec
    alp = 1;  % afterwards
elseif time > som.t_start
    alp = som.filter.alp;
end
% set en = 0 if the robot goes out of the safe envelope.
out_amp = som.filter.alp*amp + (1-som.filter.alp)*amp2;

== matlab function controller13_AIS/Vicon Measurements/MATLAB Function1 ==
  data: u input; y output
function y = fcn(u)

y = u;

== matlab function controller13_AIS/Vicon Measurements/MATLAB Function2 ==
  data: u input; y output
function y = fcn(u)

y = u;

== matlab function controller13_AIS/Vicon Measurements/MATLAB Function3 ==
  data: u input; y output
function y = fcn(u)

y = u;

== matlab function controller13_AIS/MATLAB Function2 ==
  data: u input; y output
function y = fcn(u)

y = u;

== matlab function controller13_AIS/Adaptive Controller 2/observer1/UKF/UKF_inner/UKF update then predict ==
  data: s_out output; z_raw input; z_raw_prev input; f_cmd input; tau_cmd_x input; tau_cmd_y input; s_in input; P_in_flat input; is_init_in input; sys parameter; P_out_flat output; is_init_out output
function [s_out, P_out_flat, is_init_out] = fcn(z_raw, z_raw_prev, f_cmd, tau_cmd_x, tau_cmd_y, s_in, P_in_flat, is_init_in, sys)
    [s_out, P_out_flat, is_init_out] = UKF.inner_helper(z_raw, z_raw_prev, f_cmd, tau_cmd_x, tau_cmd_y, s_in, P_in_flat, is_init_in, sys);
end

== matlab function controller13_AIS/Adaptive Controller 2/observer1/UKF/euler to quat ==
  data: euler_angles input; q output
function q = fcn(euler_angles)
% convertion from euler to R block

eu_x = euler_angles(1);
eu_y = euler_angles(2);
eu_z = euler_angles(3);

R = [cos(eu_y)*cos(eu_z); -cos(eu_y)*sin(eu_z); sin(eu_y); ...
    cos(eu_x)*sin(eu_z)+sin(eu_x)*sin(eu_y)*cos(eu_z); cos(eu_x)*cos(eu_z)-sin(eu_x)*sin(eu_y)*sin(eu_z); -sin(eu_x)*cos(eu_y); ...
    sin(eu_x)*sin(eu_z)-cos(eu_x)*sin(eu_y)*cos(eu_z); sin(eu_x)*cos(eu_z)+cos(eu_x)*sin(eu_y)*sin(eu_z); cos(eu_x)*cos(eu_y)];
% R is 1x9

R_unflattened = UKF.unflatten_matrix(R);
q = rotm2quat(R_unflattened)';
      


end

== matlab function controller13_AIS/Adaptive Controller 2/observer1/UKF/pack measurement vector ==
  data: r input; z_raw output; q input; r_dot input; omega input
function z_raw = fcn(r, q, r_dot, omega)
    z_raw = vertcat(r, q, r_dot, omega);
end

== matlab function controller13_AIS/Measurement manager 1/safety check system/landing condition/landing_cond ==
  data: alt input; en output; time_cond input; ctr1 parameter
function en = fcn(alt,time_cond,ctr1)
%#codegen
if ( (time_cond<0) | (alt>ctr1.landing.height) )
    en = 1;
else
    en = 0;
end
en=1;
end
% this lands the robot if the flight time is more than mdl.i_delay+2 and
% the robot is still on the ground.

== matlab function controller13_AIS/Adaptive Controller 2/observer1/UKF/quaternion to rotation matrix ==
  data: q input; R_flat output
function R_flat = fcn(q)
    % Assume q = [q_s; q_x, q_y, q_z];
    R = quat2rotm(q');
    R_flat = UKF.flatten_matrix(R);
end

== matlab function controller13_AIS/Adaptive Controller 2/observer1/UKF/unpack state vector ==
  data: s input; r output; q output; r_dot output; omega output
function [r, q, r_dot, omega] = fcn(s)
    [r, q, r_dot, omega] = UKF.partial_unpack_s(s);
end

== matlab function controller13_AIS/Adaptive Controller 2/observer1/UKF1/R_flat to quat ==
  data: R_flat input; q output
function q = fcn(R_flat)
% convertion from rotation matrix to quaternion
q = rotm2quat(UKF.unflatten_matrix(R_flat))';
end

== matlab function controller13_AIS/Adaptive Controller 2/observer1/UKF1/UKF_inner/UKF update then predict ==
  data: s_out output; z_raw input; z_raw_prev input; f_cmd input; tau_cmd_x input; tau_cmd_y input; s_in input; P_in_flat input; is_init_in input; s_prediction_time input; sys parameter; P_out_flat output; is_init_out output; s_out_pre output; s_prediction_out output
function [s_out, P_out_flat, is_init_out, s_out_pre, s_prediction_out] = fcn(z_raw, z_raw_prev, f_cmd, tau_cmd_x, tau_cmd_y, s_in, P_in_flat, is_init_in, s_prediction_time, sys)
    [s_out, P_out_flat, is_init_out, s_out_pre, s_prediction_out] = UKF.inner_helper(z_raw, z_raw_prev, f_cmd, tau_cmd_x, tau_cmd_y, s_in, P_in_flat, is_init_in, s_prediction_time, sys);
end

== matlab function controller13_AIS/Adaptive Controller 2/observer1/UKF1/UKF_inner/bee cov to SI cov ==
  data: P_flat_bee input; P_flat_si output
function P_flat_si  = fcn(P_flat_bee)
    P_flat_si = UKF.flatten_matrix(diag(UKF.var_bee_to_var_si(diag(UKF.unflatten_matrix(P_flat_bee)))));
end

== matlab function controller13_AIS/Adaptive Controller 2/observer1/UKF1/UKF_inner/bee units to SI ==
  data: s_bee input; s_si output
function s_si  = fcn(s_bee)
    s_si = UKF.s_bee_to_s_si(s_bee);
end

== matlab function controller13_AIS/Adaptive Controller 2/observer1/UKF1/UKF_inner/bee units to SI1 ==
  data: s_bee input; s_si output
function s_si  = fcn(s_bee)
    s_si = UKF.s_bee_to_s_si(s_bee);
end

== matlab function controller13_AIS/Adaptive Controller 2/observer1/UKF1/pack measurement vector ==
  data: r input; z_raw output; q input
function z_raw = fcn(r, q)
    z_raw = vertcat(r, q, zeros(6,1));
end

== matlab function controller13_AIS/Adaptive Controller 2/observer1/UKF1/quaternion to rotation matrix ==
  data: q input; R_flat output
function R_flat = fcn(q)
    % Assume q = [q_s; q_x, q_y, q_z];
    R = quat2rotm(q');
    R_flat = UKF.flatten_matrix(R);
end

== matlab function controller13_AIS/Adaptive Controller 2/observer1/UKF1/unpack state ==
  data: s input; r output; q output; r_dot output; omega output
function [r, q, r_dot, omega] = fcn(s)
    [r, q, r_dot, omega, ~, ~] = UKF.unpack_s(s);
end

== matlab function controller13_AIS/Adaptive Controller 1/observer/Rotaion/Rotation Matrix ==
  data: euler_angles input; R output
function R = fcn(euler_angles)
%#codegen

eu_x = euler_angles(1);
eu_y = euler_angles(2);
eu_z = euler_angles(3);

R = [cos(eu_y)*cos(eu_z); -cos(eu_y)*sin(eu_z); sin(eu_y); ...
    cos(eu_x)*sin(eu_z)+sin(eu_x)*sin(eu_y)*cos(eu_z); cos(eu_x)*cos(eu_z)-sin(eu_x)*sin(eu_y)*sin(eu_z); -sin(eu_x)*cos(eu_y); ...
    sin(eu_x)*sin(eu_z)-cos(eu_x)*sin(eu_y)*cos(eu_z); sin(eu_x)*cos(eu_z)+cos(eu_x)*sin(eu_y)*sin(eu_z); cos(eu_x)*cos(eu_y)];


end

% R is 9x1

% Pakpong was using "XYZ" convention, which seems to be the same as Vicon

== matlab function controller13_AIS/Adaptive Controller 2/observer1/UKF2/UKF_inner/UKF update then predict ==
  data: s_out output; z_raw input; z_raw_prev input; f_cmd input; tau_cmd_x input; tau_cmd_y input; s_in input; P_in_flat input; is_init_in input; sys parameter; P_out_flat output; is_init_out output
function [s_out, P_out_flat, is_init_out] = fcn(z_raw, z_raw_prev, f_cmd, tau_cmd_x, tau_cmd_y, s_in, P_in_flat, is_init_in, sys)
    [s_out, P_out_flat, is_init_out] = UKF.inner_helper(z_raw, z_raw_prev, f_cmd, tau_cmd_x, tau_cmd_y, s_in, P_in_flat, is_init_in, sys);
end

== matlab function controller13_AIS/Adaptive Controller 2/observer1/UKF2/euler to quat ==
  data: euler_angles input; q output
function q = fcn(euler_angles)
% convertion from euler to R block

eu_x = euler_angles(1);
eu_y = euler_angles(2);
eu_z = euler_angles(3);

R = [cos(eu_y)*cos(eu_z); -cos(eu_y)*sin(eu_z); sin(eu_y); ...
    cos(eu_x)*sin(eu_z)+sin(eu_x)*sin(eu_y)*cos(eu_z); cos(eu_x)*cos(eu_z)-sin(eu_x)*sin(eu_y)*sin(eu_z); -sin(eu_x)*cos(eu_y); ...
    sin(eu_x)*sin(eu_z)-cos(eu_x)*sin(eu_y)*cos(eu_z); sin(eu_x)*cos(eu_z)+cos(eu_x)*sin(eu_y)*sin(eu_z); cos(eu_x)*cos(eu_y)];
% R is 1x9

R_unflattened = UKF.unflatten_matrix(R);
q = rotm2quat(R_unflattened)';
      


end

== matlab function controller13_AIS/Adaptive Controller 2/observer1/UKF2/pack measurement vector ==
  data: r input; z_raw output; q input; r_dot input; omega input
function z_raw = fcn(r, q, r_dot, omega)
    z_raw = vertcat(r, q, r_dot, omega);
end

== matlab function controller13_AIS/Adaptive Controller 2/observer1/UKF2/quaternion to rotation matrix ==
  data: q input; R_flat output
function R_flat = fcn(q)
    % Assume q = [q_s; q_x, q_y, q_z];
    R = quat2rotm(q');
    R_flat = UKF.flatten_matrix(R);
end

== matlab function controller13_AIS/Adaptive Controller 2/observer1/UKF2/unpack state vector ==
  data: s input; r output; q output; r_dot output; omega output
function [r, q, r_dot, omega] = fcn(s)
    [r, q, r_dot, omega] = UKF.partial_unpack_s(s);
end

== matlab function controller13_AIS/Adaptive Controller 2/observer1/eul to rotation matrix ==
  data: euler_angles input; R output
function R = fcn(euler_angles)
%#codegen

eu_x = euler_angles(1);
eu_y = euler_angles(2);
eu_z = euler_angles(3);

R = [cos(eu_y)*cos(eu_z); -cos(eu_y)*sin(eu_z); sin(eu_y); ...
    cos(eu_x)*sin(eu_z)+sin(eu_x)*sin(eu_y)*cos(eu_z); cos(eu_x)*cos(eu_z)-sin(eu_x)*sin(eu_y)*sin(eu_z); -sin(eu_x)*cos(eu_y); ...
    sin(eu_x)*sin(eu_z)-cos(eu_x)*sin(eu_y)*cos(eu_z); sin(eu_x)*cos(eu_z)+cos(eu_x)*sin(eu_y)*sin(eu_z); cos(eu_x)*cos(eu_y)];
% R is 1x9 (actually 9x1)
% euler_angles: assuming r, p, y
% euler_angles = euler_angles(:)';
% R = eul2rotm(euler_angles);
end

== matlab function controller13_AIS/MATLAB Function3 ==
  data: u input; y output
function y = fcn(u)

y = u;

== matlab function controller13_AIS/Adaptive Controller 1/attitude and thrust controller/Thrust Controller ==
  data: r input; F output size=1; r_dot input; r_dotdot input; R input; Omega input; rd input; rd_d input; rd_dd input; rd_ddd input; rd_dddd input; int_e input; mdl parameter; alt_e output size=1; ctr1 parameter
function [F, alt_e] = fcn(r, r_dot, r_dotdot, R, Omega, rd,rd_d,rd_dd,rd_ddd,rd_dddd, int_e, mdl, ctr1)
%#codegen

%% init
R11 = R(1);
R12 = R(2);
R13 = R(3);
R21 = R(4);
R22 = R(5);
R23 = R(6);
R31 = R(7);
R32 = R(8);
R33 = R(9);

% feedforward
% -> (0m, 0) -> (0.1m, 0.2)
ffwd = mdl.g * max(0,(rd(3)*1.25-0.02));

F = rd_dd(3) - ctr1.gain.al1*( r_dot(3)-rd_d(3) ) - ctr1.gain.al0*( r(3)-rd(3) );
% F = 0 - ctr.gain.al1*( r_dot(3)) - ctr.gain.al0*( r(3)-ctr.setpoint.z );
F = mdl.g + F + ctr1.gain.ali*int_e(4) + ffwd; % g + control + integral + feedforward
F = F/R33;
F = max(min(F, mdl.g+4), mdl.g-4.0); % during hovering.

alt_e = -( r(3)-rd(3) )/R33;
% alt_e = -( r(3)- ctr.setpoint.z )/R33;
end
